simulink model "bike_rider_model"  (R2018b)
settings: Solver=VariableStepAuto  StartTime=0.0  StopTime=10.0  RelTol=1e-3
undefined symbols (not defined in the file or in its folder): G11_den, G11_num, G12_den, G12_num, G21_den, G21_num, G22_den, G22_num
libraries: dspsrcs4 x1
settings Model: Creator=chris  LastModifiedBy=chris

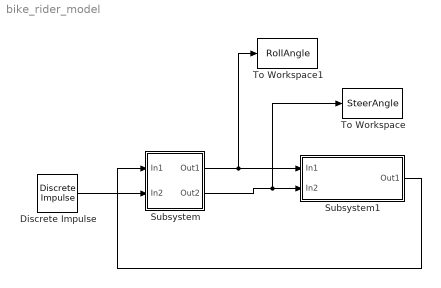
== system bike_rider_model ==
  Discrete Impulse : dspsrcs4/Discrete  Impulse  Delay=0  SampleTime=1  FrameSample=1  OutputFrames=off  dataType=double  isSigned=on  wordLen=16  udDataType=sfix(16)  fracBitsMode=Best precision  numFracBits=15  OutDataTypeStr=double  LastOutDataTypeStr=double
  Subsystem : Subsystem
  Subsystem1 : Subsystem
  To Workspace : ToWorkspace  VariableName=SteerAngle  SaveFormat=Timeseries  SampleTime=-1
  To Workspace1 : ToWorkspace  VariableName=RollAngle  SaveFormat=Timeseries  SampleTime=-1
  wires:
  Subsystem/2(Out2) -> To Workspace/1, Subsystem1/2(In2)
  Subsystem/1(Out1) -> To Workspace1/1, Subsystem1/1(In1)
  Subsystem1/1(Out1) -> Subsystem/1(In1)
  Discrete Impulse/1 -> Subsystem/2(In2)

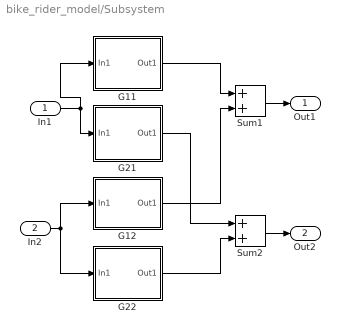
== system bike_rider_model/Subsystem ==
  In1 : Inport
  In2 : Inport  Port=2
  G11 : Subsystem
  G12 : Subsystem
  G21 : Subsystem
  G22 : Subsystem
  Sum1 : Sum  SaturateOnIntegerOverflow=on  InputSameDT=on  OutDataTypeStr=Inherit: Same as first input
  Sum2 : Sum  SaturateOnIntegerOverflow=on  InputSameDT=on  OutDataTypeStr=Inherit: Same as first input
  Out1 : Outport  InitialOutput=0
  Out2 : Outport  Port=2  InitialOutput=0
  wires:
  In1/1 -> G11/1(In1), G21/1(In1)
  G21/1(Out1) -> Sum2/1
  G12/1(Out1) -> Sum1/2
  G11/1(Out1) -> Sum1/1
  G22/1(Out1) -> Sum2/2
  In2/1 -> G12/1(In1), G22/1(In1)
  Sum1/1 -> Out1/1
  Sum2/1 -> Out2/1

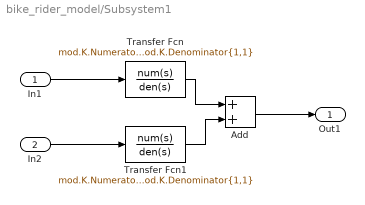
== system bike_rider_model/Subsystem1 ==
  In1 : Inport
  In2 : Inport  Port=2
  Add : Sum
  Transfer Fcn : TransferFcn  Numerator=mod.K.Numerator{1,1}  Denominator=mod.K.Denominator{1,1}
  Transfer Fcn1 : TransferFcn  Numerator=mod.K.Numerator{1,1}  Denominator=mod.K.Denominator{1,1}
  Out1 : Outport
  wires:
  In1/1 -> Transfer Fcn/1
  Transfer Fcn/1 -> Add/1
  Transfer Fcn1/1 -> Add/2
  In2/1 -> Transfer Fcn1/1
  Add/1 -> Out1/1

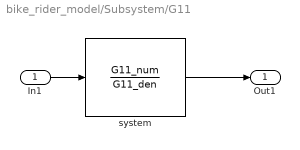
== system bike_rider_model/Subsystem/G11 ==
  In1 : Inport
  system : TransferFcn  Numerator=G11_num  Denominator=G11_den
  Out1 : Outport  InitialOutput=0
  wires:
  In1/1 -> system/1
  system/1 -> Out1/1

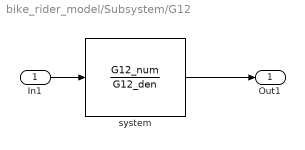
== system bike_rider_model/Subsystem/G12 ==
  In1 : Inport
  system : TransferFcn  Numerator=G12_num  Denominator=G12_den
  Out1 : Outport  InitialOutput=0
  wires:
  In1/1 -> system/1
  system/1 -> Out1/1

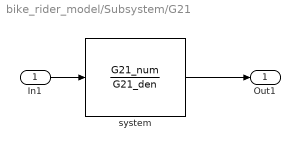
== system bike_rider_model/Subsystem/G21 ==
  In1 : Inport
  system : TransferFcn  Numerator=G21_num  Denominator=G21_den
  Out1 : Outport  InitialOutput=0
  wires:
  In1/1 -> system/1
  system/1 -> Out1/1

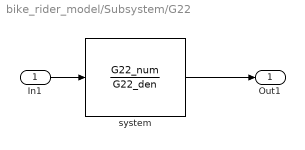
== system bike_rider_model/Subsystem/G22 ==
  In1 : Inport
  system : TransferFcn  Numerator=G22_num  Denominator=G22_den
  Out1 : Outport  InitialOutput=0
  wires:
  In1/1 -> system/1
  system/1 -> Out1/1
